simulink model "Check_my_Aerodynamics"  (R2020b)
settings: Solver=FixedStepAuto  StartTime=0.0  StopTime=100  FixedStep=CNT_StepSize  RelTol=1e-3
undefined symbols (not defined in the file): Aerodynamics
settings Model: Creator=NicolasS  LastModifiedBy=NicolasS

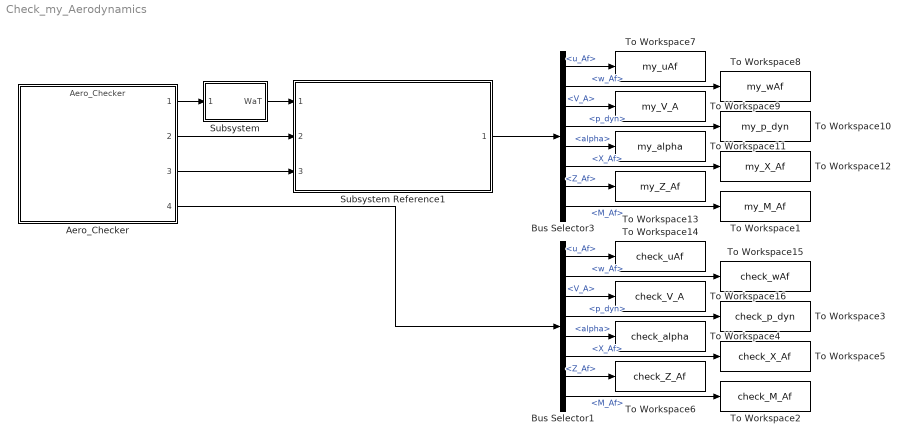
== system Check_my_Aerodynamics ==
  Aero_Checker : ModelReference  ModelNameDialog=Aero_Checker.slxp  UsingDefaultArgumentValue=0,0,0,0,0,0,0,0,0,0,0,0,0  ModelReferenceVersion=1.21  CopyOfModelProtected=on  C_X0=-Aerodynamics.Ca_D0  C_Xa=Aerodynamics.Ca_L0 - Aerodynamics.Ca_Da  C_Xa2=Aerodynamics.Ca_La - Aerodynamics.Ca_Da2  C_Z0=-Aerodynamics.Ca_L0  C_Za=-Aerodynamics.Ca_La - Aerodynamics.Ca_D0  C_Zq=-Aerodynamics.Ca_Lq  C_Zde=-Aerodynamics.Ca_Lde  C_m0=Aerodynamics.Ca_m0  C_ma=Aerodynamics.Ca_ma  C_mde=Aerodynamics.Ca_mde  C_mq=Aerodynamics.Ca_mq  S=Aerodynamics.S  cbar=Aerodynamics.cbar
  Bus Selector1 : BusSelector  OutputSignals=AirData.u_Af,AirData.w_Af,AirData.V_A,AirData.p_dyn,AirData.alpha,X_Af,Z_Af,M_Af
  Bus Selector3 : BusSelector  OutputSignals=AirData.u_Af,AirData.w_Af,AirData.V_A,AirData.p_dyn,AirData.alpha,X_Af,Z_Af,M_Af
  Subsystem : Subsystem
  Subsystem Reference1 : Subsystem  ReferencedSubsystem=Aerodyn
  To Workspace1 : ToWorkspace  VariableName=my_M_Af  SaveFormat=Timeseries  SampleTime=-1
  To Workspace10 : ToWorkspace  VariableName=my_p_dyn  SaveFormat=Timeseries  SampleTime=-1
  To Workspace11 : ToWorkspace  VariableName=my_alpha  SaveFormat=Timeseries  SampleTime=-1
  To Workspace12 : ToWorkspace  VariableName=my_X_Af  SaveFormat=Timeseries  SampleTime=-1
  To Workspace13 : ToWorkspace  VariableName=my_Z_Af  SaveFormat=Timeseries  SampleTime=-1
  To Workspace14 : ToWorkspace  VariableName=check_uAf  SaveFormat=Timeseries  SampleTime=-1
  To Workspace15 : ToWorkspace  VariableName=check_wAf  SaveFormat=Timeseries  SampleTime=-1
  To Workspace16 : ToWorkspace  VariableName=check_V_A  SaveFormat=Timeseries  SampleTime=-1
  To Workspace2 : ToWorkspace  VariableName=check_M_Af  SaveFormat=Timeseries  SampleTime=-1
  To Workspace3 : ToWorkspace  VariableName=check_p_dyn  SaveFormat=Timeseries  SampleTime=-1
  To Workspace4 : ToWorkspace  VariableName=check_alpha  SaveFormat=Timeseries  SampleTime=-1
  To Workspace5 : ToWorkspace  VariableName=check_X_Af  SaveFormat=Timeseries  SampleTime=-1
  To Workspace6 : ToWorkspace  VariableName=check_Z_Af  SaveFormat=Timeseries  SampleTime=-1
  To Workspace7 : ToWorkspace  VariableName=my_uAf  SaveFormat=Timeseries  SampleTime=-1
  To Workspace8 : ToWorkspace  VariableName=my_wAf  SaveFormat=Timeseries  SampleTime=-1
  To Workspace9 : ToWorkspace  VariableName=my_V_A  SaveFormat=Timeseries  SampleTime=-1
  wires:
  Aero_Checker/2 -> Subsystem Reference1/2
  Aero_Checker/3 -> Subsystem Reference1/3
  Bus Selector3/7 -> To Workspace13/1  "<Z_Af>"
  Aero_Checker/4 -> Bus Selector1/1
  Bus Selector3/2 -> To Workspace8/1  "<w_Af>"
  Bus Selector3/6 -> To Workspace12/1  "<X_Af>"
  Bus Selector3/3 -> To Workspace9/1  "<V_A>"
  Bus Selector3/1 -> To Workspace7/1  "<u_Af>"
  Bus Selector3/5 -> To Workspace11/1  "<alpha>"
  Bus Selector3/4 -> To Workspace10/1  "<p_dyn>"
  Subsystem Reference1/1 -> Bus Selector3/1
  Bus Selector3/8 -> To Workspace1/1  "<M_Af>"
  Bus Selector1/4 -> To Workspace3/1  "<p_dyn>"
  Bus Selector1/8 -> To Workspace2/1  "<M_Af>"
  Bus Selector1/7 -> To Workspace6/1  "<Z_Af>"
  Bus Selector1/5 -> To Workspace4/1  "<alpha>"
  Bus Selector1/1 -> To Workspace14/1  "<u_Af>"
  Bus Selector1/6 -> To Workspace5/1  "<X_Af>"
  Bus Selector1/2 -> To Workspace15/1  "<w_Af>"
  Bus Selector1/3 -> To Workspace16/1  "<V_A>"
  Aero_Checker/1 -> Subsystem/1(WaT_in)
  Subsystem/1(WaT) -> Subsystem Reference1/1

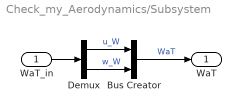
== system Check_my_Aerodynamics/Subsystem ==
  WaT_in : Inport
  Bus Creator : BusCreator  Inputs=2  OutDataTypeStr=Bus: WaT
  Demux : Demux  Outputs=2
  WaT : Outport
  wires:
  Demux/1 -> Bus Creator/1  "u_W"
  WaT_in/1 -> Demux/1
  Demux/2 -> Bus Creator/2  "w_W"
  Bus Creator/1 -> WaT/1  "WaT"
